simulink model "closed_loop_step"  (R2023b)
settings: Solver=ode4  StartTime=0.0  StopTime=Inf  FixedStep=0.001  RelTol=1e-3  EnableMultiTasking=on
undefined symbols (not defined in the file): k_i, k_p, National_Instruments, PCI
libraries: sldrtlib x2
settings Model: SimulationMode=external  ExtModeTrigDuration=300000  ExtModeTrigDurationFloating=300  ExtModeArchiveFileName=Arm motion with Impulse  ExtModeArchiveDirName=E:\work\test1\NachumEisen\Exp1  Creator=test1  LastModifiedBy=me-int1
settings SolverCC: AlgebraicLoopSolver=TrustRegion
settings DataIOCC: SaveFormat=Array  ReturnWorkspaceOutputs=off
settings DebuggingCC: UnconnectedInputMsg=warning  UnconnectedOutputMsg=warning  UnconnectedLineMsg=warning  SFUnexpectedBacktrackingDiag=warning  SFNoUnconditionalDefaultTransitionDiag=warning  SFExecutionAtInitializationDiag=none  ArithmeticOperatorsInVariantConditions=warning
settings HardwareCC: ProdBitPerLong=64  ProdHWDeviceType=Intel->x86-64 (Linux 64)  TargetBitPerLong=64  TargetBitPerPointer=64  TargetIntDivRoundTo=Zero  TargetEndianess=LittleEndian  TargetWordSize=64  TargetHWDeviceType=Intel->x86-64
settings ModelReferenceCC: EnableRefExpFcnMdlSchedulingChecks=on  PropagateSignalLabelsOutOfModel=off
settings SFSimCC: SimUseLocalCustomCode=off  CustomCodeUndefinedFunction=UseInterfaceOnly
settings RTWCC: Description=Simulink Desktop Real-Time  SystemTargetFile=sldrt.tlc  TemplateMakefile=sldrt.tmf  RTWUseLocalCustomCode=off  RTWCompilerOptimization=on
settings CodeAppCC: MaxIdLength=95  StateflowObjectComments=on
settings SimulinkDesktopRealTimeCC: TargetLibSuffix=_sldrt.a  TargetPreCompLibLocation=C:\Program Files\MATLAB\R2023b\toolbox\sldrt\lib\win64  TargetLangStandard=C89/C90 (ANSI)  SupportVariableSizeSignals=off
settings ConfigComp: CovMetricSettings=dw  CovSaveCumulativeToWorkspaceVar=on  CovSaveSingleToWorkspaceVar=on  CovExternalEMLEnable=off

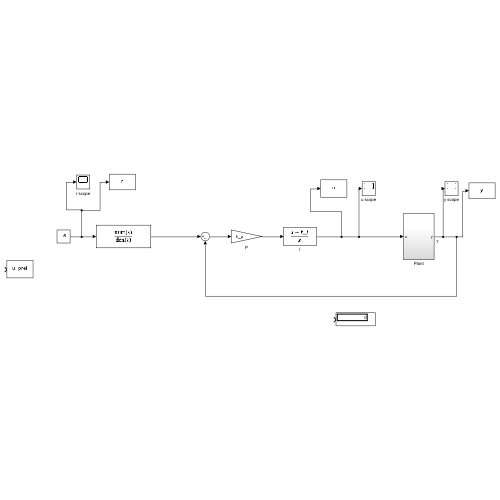
[thumbnail: Simulink's stored preview of the top-level diagram]
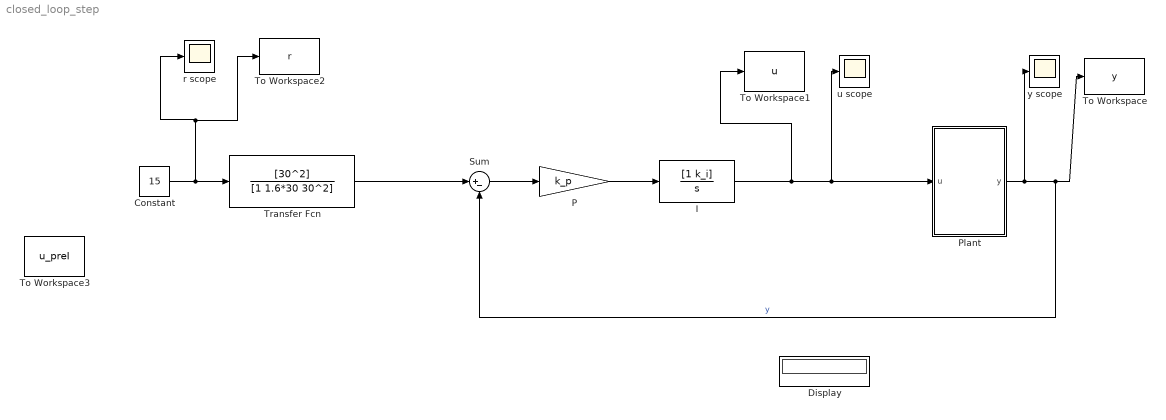
== system closed_loop_step ==
  Constant : Constant  Value=15
  Display : Display
  I : TransferFcn  Numerator=[1 k_i]  Denominator=[1 0]
  P : Gain  Gain=k_p
  Plant : Subsystem
  Sum : Sum  Inputs=|+-
  To Workspace : ToWorkspace  VariableName=y  SaveFormat=Structure With Time  SampleTime=-1
  To Workspace1 : ToWorkspace  VariableName=u  SaveFormat=Structure With Time  SampleTime=-1
  To Workspace2 : ToWorkspace  VariableName=r  SaveFormat=Structure With Time  SampleTime=-1
  To Workspace3 : ToWorkspace  VariableName=u_preI  SaveFormat=Structure With Time  SampleTime=-1
  Transfer Fcn : TransferFcn  Numerator=[30^2]  Denominator=[1 1.6*30 30^2]
  r scope : Scope
  u scope : Scope
  y scope : Scope
  wires:
  Constant/1 -> To Workspace2/1, r scope/1, Transfer Fcn/1
  Sum/1 -> P/1
  Plant/1(y) -> To Workspace/1, Sum/2, y scope/1  "y"
  Transfer Fcn/1 -> Sum/1
  I/1 -> To Workspace1/1, u scope/1, Plant/1(u)
  P/1 -> I/1

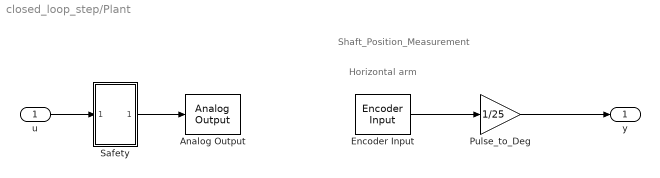
== system closed_loop_step/Plant ==
  note: Shaft_Position_Measurement
  note: Horizontal arm
  u : Inport
  Analog Output : sldrtlib/Analog Output  SampleTime=0.001  MaxMissedTicks=10  ShowMissedTicks=off  YieldWhenWaiting=off  DrvName=National_Instruments/PCI-6221  DrvAddress=4294967295  DrvOptions=[0 0 0 2 2]  Channels=[2]  RangeMode=1  VoltRange=1  InitialValue=0  FinalValue=0
      settings: AttributesFormatString=National Instruments\nPCI-6221 [auto]
  Encoder Input : sldrtlib/Encoder Input  SampleTime=0.001  MaxMissedTicks=10  ShowMissedTicks=off  YieldWhenWaiting=off  DrvName=National_Instruments/PCI-6221  DrvAddress=4294967295  DrvOptions=[0 0 0 2 2]  Channels=[1]  QuadMode=3  IndexPulse=1  InputFilter=Inf  DataType=1
      settings: AttributesFormatString=National Instruments\nPCI-6221 [auto]
  Pulse_to_Deg : Gain  Gain=1/25
  Safety : Subsystem
  y : Outport
  wires:
  u/1 -> Safety/1(In1)
  Pulse_to_Deg/1 -> y/1
  Safety/1(Out1) -> Analog Output/1
  Encoder Input/1 -> Pulse_to_Deg/1

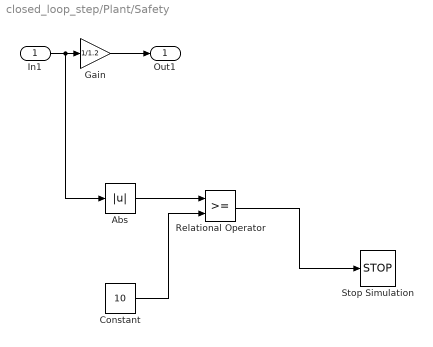
== system closed_loop_step/Plant/Safety ==
  In1 : Inport
  Abs : Abs  SaturateOnIntegerOverflow=off
  Constant : Constant  Value=10
  Gain : Gain  Gain=1/1.2
  Relational Operator : RelationalOperator  OutDataTypeStr=boolean  InputSameDT=off
  Stop Simulation : Stop
  Out1 : Outport
  wires:
  In1/1 -> Abs/1, Gain/1
  Gain/1 -> Out1/1
  Relational Operator/1 -> Stop Simulation/1
  Constant/1 -> Relational Operator/2
  Abs/1 -> Relational Operator/1
